simulink subsystem "thrust_control_sub"  (R2025b)
settings: Solver=VariableStepAuto  StartTime=0.0  StopTime=10.0  RelTol=1e-3
libraries: slpidlib x1
settings Model: Creator=lew11  LastModifiedBy=lew11

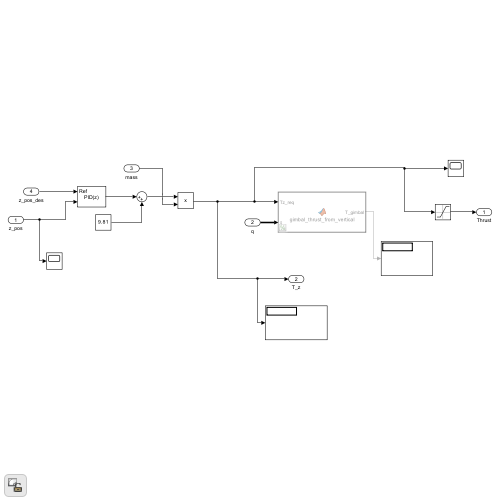
[thumbnail: Simulink's stored preview of the top-level diagram]
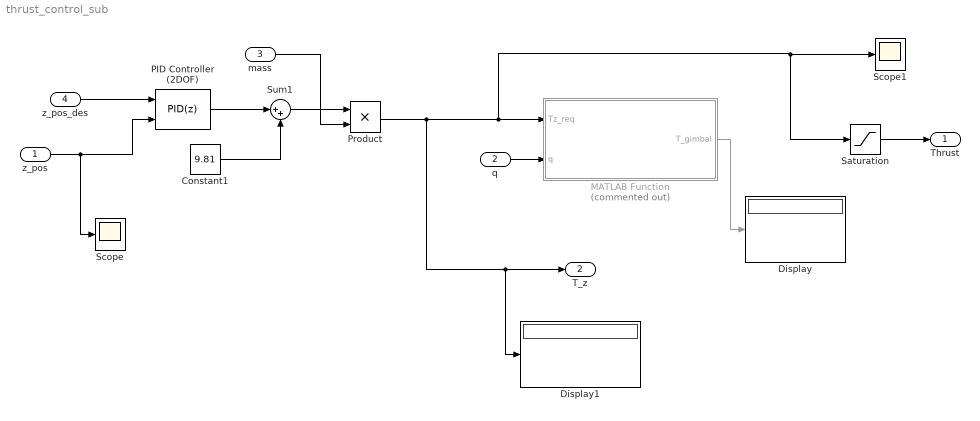
== system thrust_control_sub ==
  z_pos : Inport
  q : Inport  Port=2  PortDimensions=4
  mass : Inport  Port=3
  z_pos_des : Inport  Port=4  PortDimensions=1
  Constant1 : Constant  Value=9.81
  Display : Display
  Display1 : Display
  MATLAB Function : MATLAB Function  Commented=on  TreatAsAtomicUnit=on
  PID Controller (2DOF) : slpidlib/PID Controller (2DOF)  Controller=PID  Form=Parallel  TimeDomain=Discrete-time  UseExternalTs=off  SampleTime=-1  IntegratorMethod=Forward Euler  FilterMethod=Forward Euler  ControllerParametersSource=internal  P=0.157147988939319  I=0.00595653688310268  UseKiTs=off  D=0.992186991424612  UseExternalDerivativeSource=off  N=114.28279760416  UseFilter=on  b=1  c=1  TunerSelectOption=Transfer Function Based (PID Tuner App)  InitialConditionSource=internal  InitialConditionForIntegrator=0  InitialConditionForFilter=0  DifferentiatorICPrevScaledInput=0  ExternalReset=none  TrackingMode=off  Kt=1  LimitOutput=off  SatLimitsSource=internal  UpperSaturationLimit=inf  LowerSaturationLimit=-inf  LinearizeAsGain=on  AntiWindupMode=none  Kb=1  LimitIntegrator=off  UpperIntegratorSaturationLimit=inf  LowerIntegratorSaturationLimit=-inf  POutMin=[]  POutMax=[]  IOutMin=[]  IOutMax=[]  DOutMin=[]  DOutMax=[]  NOutMin=[]  NOutMax=[]  bOutMin=[]  bOutMax=[]  cOutMin=[]  cOutMax=[]  SumOutMin=[]  SumOutMax=[]  SaturationOutMin=[]  SaturationOutMax=[]  PParamMin=[]  PParamMax=[]  IParamMin=[]  IParamMax=[]  DParamMin=[]  DParamMax=[]  NParamMin=[]  NParamMax=[]  bParamMin=[]  bParamMax=[]  cParamMin=[]  cParamMax=[]  KbParamMin=[]  KbParamMax=[]  KtParamMin=[]  KtParamMax=[]  KbOutMin=[]  KbOutMax=[]  KtOutMin=[]  KtOutMax=[]  IntegratorOutMin=[]  IntegratorOutMax=[]  FilterOutMin=[]  FilterOutMax=[]  SumI1OutMin=[]  SumI1OutMax=[]  SumI2OutMin=[]  SumI2OutMax=[]  SumI3OutMin=[]  SumI3OutMax=[]  SumI4OutMin=[]  SumI4OutMax=[]  SumDOutMin=[]  SumDOutMax=[]  Sum1OutMin=[]  Sum1OutMax=[]  Sum2OutMin=[]  Sum2OutMax=[]  Sum3OutMin=[]  Sum3OutMax=[]  DifferentiatorOutMin=[]  DifferentiatorOutMax=[]  FilterDiffOutCoefMin=[]  FilterDiffOutCoefMax=[]  ReciprocalOutMin=[]  ReciprocalOutMax=[]  SumDenOutMin=[]  SumDenOutMax=[]  SumNumOutMin=[]  SumNumOutMax=[]  DivideOutMin=[]  DivideOutMax=[]  UdiffTsProdOutMin=[]  UdiffTsProdOutMax=[]  NTsProdOutMin=[]  NTsProdOutMax=[]  UintegralTsProdOutMin=[]  UintegralTsProdOutMax=[]  UngainTsProdOutMin=[]  UngainTsProdOutMax=[]  ClampingZeroOutDataTypeStr=Inherit: Inherit via back propagation  ClampingZeroOutMin=[]  ClampingZeroOutMax=[]  FilterDenConstantOutDataTypeStr=Inherit: Inherit via back propagation  FilterDenConstantOutMin=[]  FilterDenConstantOutMax=[]  PCopyOutDataTypeStr=Inherit: Inherit via back propagation  PCopyOutMin=[]  PCopyOutMax=[]  NCopyOutDataTypeStr=Inherit: Inherit via back propagation  NCopyOutMin=[]  NCopyOutMax=[]  IntegratorContinuousStateAttributes=''  IntegratorStateMustResolveToSignalObject=off  IntegratorRTWStateStorageClass=Auto  FilterContinuousStateAttributes=''  FilterStateMustResolveToSignalObject=off  FilterRTWStateStorageClass=Auto  ParallelPVariant=InternalParameters  IdealPVariant=Disabled  IVariant=InternalParameters  DVariant=InternalParameters  bVariant=InternalParameters  cVariant=InternalParameters  IntegratorVariant=Discrete  SatVariant=Disabled  AWVariant=Passthrough  PCopyVariant=Disabled  TRVariant=Disabled  FdbkBlocksVariant=Forward  IdealPFdbkVariant=Disabled  SatFdbkVariant=Disabled  DerivativeFilterVariant=ForwardEulerFilter  NVariant=InternalParameters  NCopyVariant=Disabled  FilterICVariant=InternalICsFilter  IntegratorICVariant=InternalICs  ExternalResetVariant=Disabled  TRSumVariant=Passthrough  SumFdbkVariant=Disabled  SumVariant=Sum_PID  TsampFilterVariant=InternalTs  TsampNgainVariant=Passthrough  TsampIntegralVariant=Disabled_SignalSpec  ExternalSaturationOutDataTypeStr=Inherit: Same as second input  DerivativeSourceVariant=ErrorSignal  PreIntVariant=InternalPreInt
  Product : Product
  Saturation : Saturate  UpperLimit=30  LowerLimit=10
  Scope : Scope
      settings: ActiveDisplayYMinimum=-2001.4047615524587  ActiveDisplayYMaximum=102.82451027803836  DataLoggingVariableName=ScopeData3
  Scope1 : Scope
      settings: ActiveDisplayYMinimum=-8.1092064892693166E+75  ActiveDisplayYMaximum=6.7677643509326E+76  DataLoggingVariableName=ScopeData12
  Sum1 : Sum  Inputs=|++
  Thrust : Outport
  T_z : Outport  Port=2
  wires:
  Saturation/1 -> Thrust/1
  Constant1/1 -> Sum1/2
  z_pos/1 -> Scope/1, PID Controller (2DOF)/2
  q/1 -> MATLAB Function/2(q)
  mass/1 -> Product/2
  PID Controller (2DOF)/1 -> Sum1/1
  Sum1/1 -> Product/1
  MATLAB Function/1(T_gimbal) -> Display/1
  z_pos_des/1 -> PID Controller (2DOF)/1
  Product/1 -> Scope1/1, Saturation/1, MATLAB Function/1(Tz_req), T_z/1, Display1/1

== matlab function thrust_control_sub/MATLAB Function ==
  data: Tz_req input; T_gimbal output; q input
function T_gimbal = gimbal_thrust_from_vertical(Tz_req, q)
% q = [qw qx qy qz], body->world, normalized

qx = q(2);
qy = q(3);

cosTilt = 1 - 2*(qx^2 + qy^2);   % = R33

% Protect against near-90deg tilt (cos -> 0)
cosMin = 0.1;                    % choose (e.g., limits to ~84 deg)
cosEff = max(cosTilt, cosMin);

T_gimbal = Tz_req / cosEff;
